simulink model "domaci2s"  (R2024b)
settings: Solver=VariableStepAuto  StartTime=0.0  StopTime=10.0  RelTol=1e-3
settings Model: Creator=neso  LastModifiedBy=neso

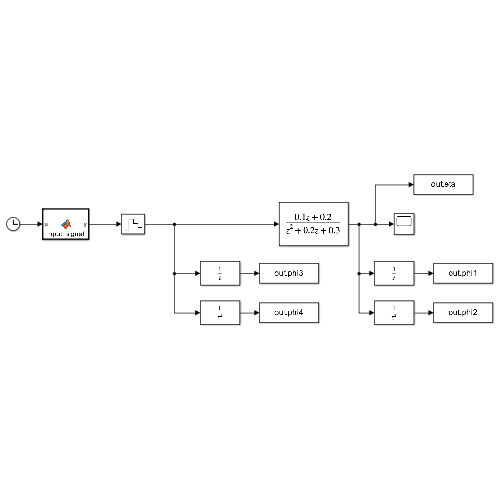
[thumbnail: Simulink's stored preview of the top-level diagram]
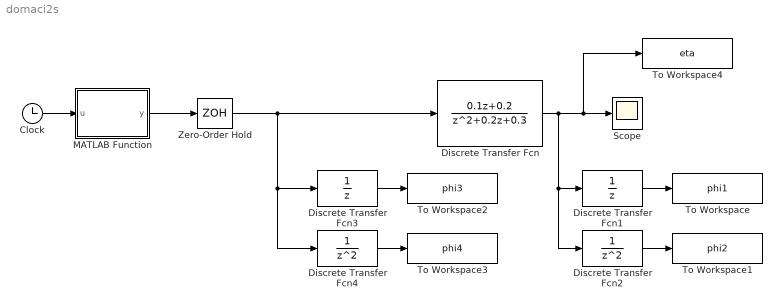
== system domaci2s ==
  Clock : Clock
  Discrete Transfer Fcn : DiscreteTransferFcn  Numerator=[0.1, 0.2]  Denominator=[1, 0.2, 0.3]
  Discrete Transfer Fcn1 : DiscreteTransferFcn  Denominator=[1, 0]
  Discrete Transfer Fcn2 : DiscreteTransferFcn  Denominator=[1, 0, 0]
  Discrete Transfer Fcn3 : DiscreteTransferFcn  Denominator=[1, 0]
  Discrete Transfer Fcn4 : DiscreteTransferFcn  Denominator=[1, 0, 0]
  MATLAB Function : MATLAB Function  TreatAsAtomicUnit=on
  Scope : Scope
  To Workspace : ToWorkspace  VariableName=phi1  SaveFormat=Timeseries  SampleTime=-1
  To Workspace1 : ToWorkspace  VariableName=phi2  SaveFormat=Timeseries  SampleTime=-1
  To Workspace2 : ToWorkspace  VariableName=phi3  SaveFormat=Timeseries  SampleTime=-1
  To Workspace3 : ToWorkspace  VariableName=phi4  SaveFormat=Timeseries  SampleTime=-1
  To Workspace4 : ToWorkspace  VariableName=eta  SaveFormat=Timeseries  SampleTime=-1
  Zero-Order Hold : ZeroOrderHold  SampleTime=0.01
  wires:
  Discrete Transfer Fcn/1 -> Discrete Transfer Fcn2/1, Discrete Transfer Fcn1/1, To Workspace4/1, Scope/1
  Zero-Order Hold/1 -> Discrete Transfer Fcn3/1, Discrete Transfer Fcn4/1, Discrete Transfer Fcn/1
  Clock/1 -> MATLAB Function/1(u)
  Discrete Transfer Fcn1/1 -> To Workspace/1
  Discrete Transfer Fcn2/1 -> To Workspace1/1
  Discrete Transfer Fcn4/1 -> To Workspace3/1
  Discrete Transfer Fcn3/1 -> To Workspace2/1
  MATLAB Function/1(y) -> Zero-Order Hold/1

== matlab function domaci2s/MATLAB Function ==
  data: u input; y output
function y = input_signal(u)
    y = 0;
    f = 0.1;
    for i = 1:100
        y = y + sin(2 * pi * i * f * u);
    end
end
